simulink model "overall_model"  (R2025b)
settings: Solver=VariableStepAuto  StartTime=0.0  StopTime=10.0  RelTol=1e-3
undefined symbols (not defined in the file): mu, r0, v0
settings Model: Creator=jennaparker  LastModifiedBy=jennaparker

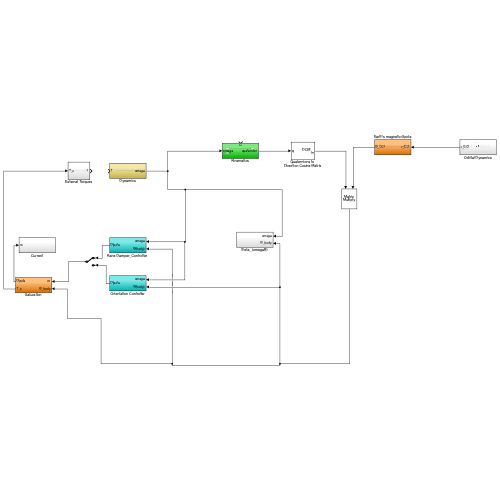
[thumbnail: Simulink's stored preview of the top-level diagram]
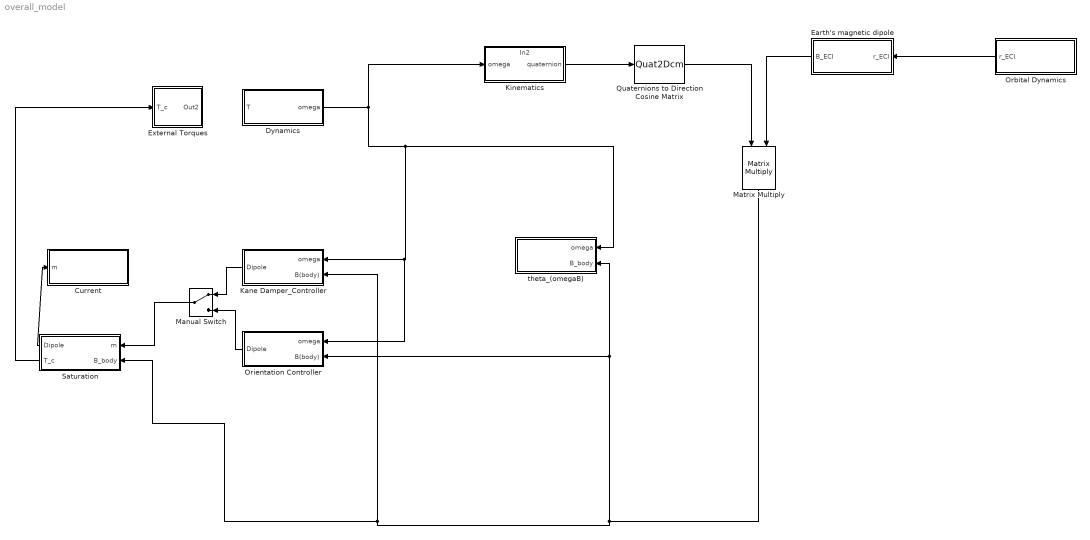
== system overall_model ==
  Current : Subsystem
  Dynamics : Subsystem
  Earth's magnetic dipole : Subsystem
  External Torques : Subsystem
  "Kane Damper_Controller " : Subsystem
  Kinematics : Subsystem
      settings: PortSchema="{\"entries\":[{\"content\":{\"sides\":[{\"content\":{\"connectorIds\":[\"In1\"]},\"type\":\"ConnectorPlacement.EquallySpacedRectSide\",\"uuid\":\"f969ea70-541e-4fe1-872d-de061585d56f\"},{\"content\":{\"connectorIds\":[\"Out1\"],\"side\":\"RIGHT\"},\"type\":\"ConnectorPlacement.EquallySpacedRectSide\",\"uuid\":\"eedb882a-61c8-46fc-b7af-f3b92c7e034c\"},{\"content\":{\"connectorIds\":[\"In2\"],\"side\":\"TOP\"},\"type\":\"ConnectorPlacement.EquallySpacedRectSide\",\"uuid\":\"40921da9-8314-4e61-b07a-c2869347cf07\"}]},\"type\":\"ConnectorPlacement.EquallySpacedConnector\",\"uuid\":\"ff868737-3a70-487e-8d9f-1b62f4bfbdd1\"}],\"packageUris\":[\"http://schema.mathworks.com/mf0/Connector/R2020b\"],\"version\":\"1.0\"}"
  Manual Switch : ManualSwitch
  Matrix Multiply : Product  Multiplication=Matrix(*)
  Orbital Dynamics : Subsystem
  Orientation Controller : Subsystem
  Quaternions to Direction Cosine Matrix : Quat2Dcm
  Saturation : Subsystem
  theta_(omegaB) : Subsystem
  wires:
  Orbital Dynamics/1(r_ECI) -> Earth's magnetic dipole/1(r_ECI)
  Earth's magnetic dipole/1(B_ECI) -> Matrix Multiply/2
  Quaternions to Direction Cosine Matrix/1 -> Matrix Multiply/1
  Kinematics/1(quaternion) -> Quaternions to Direction Cosine Matrix/1
  Dynamics/1(omega) -> Orientation Controller/1(omega), "Kane Damper_Controller "/1(omega), theta_(omegaB)/1(omega), Kinematics/1(omega)
  Saturation/1(Dipole) -> Current/1("m ")
  Saturation/2(T_c) -> External Torques/1(T_c)
  "Kane Damper_Controller "/1(Dipole) -> Manual Switch/1
  Orientation Controller/1(Dipole) -> Manual Switch/2
  Manual Switch/1 -> Saturation/1(m)
  Matrix Multiply/1 -> "Kane Damper_Controller "/2(B(body)), Saturation/2(B_body), Orientation Controller/2(B(body)), theta_(omegaB)/2(B_body)

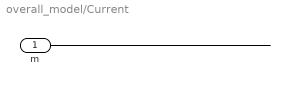
== system overall_model/Current ==
  "m " : Inport
  wires:
  "m "/1 -> ?

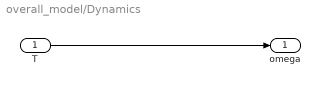
== system overall_model/Dynamics ==
  T : Inport
  omega : Outport
  wires:
  T/1 -> omega/1

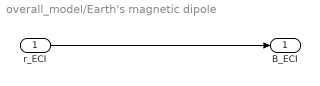
== system overall_model/Earth's magnetic dipole ==
  r_ECI : Inport
  B_ECI : Outport
  wires:
  r_ECI/1 -> B_ECI/1

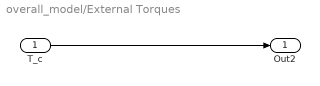
== system overall_model/External Torques ==
  T_c : Inport
  Out2 : Outport
  wires:
  T_c/1 -> Out2/1

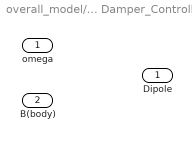
== system overall_model/Kane Damper_Controller  ==
  omega : Inport
  B(body) : Inport  Port=2
  Dipole : Outport

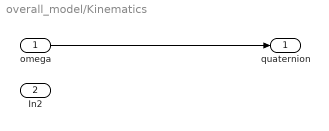
== system overall_model/Kinematics ==
  omega : Inport
  In2 : Inport  Port=2
  quaternion : Outport
  wires:
  omega/1 -> quaternion/1

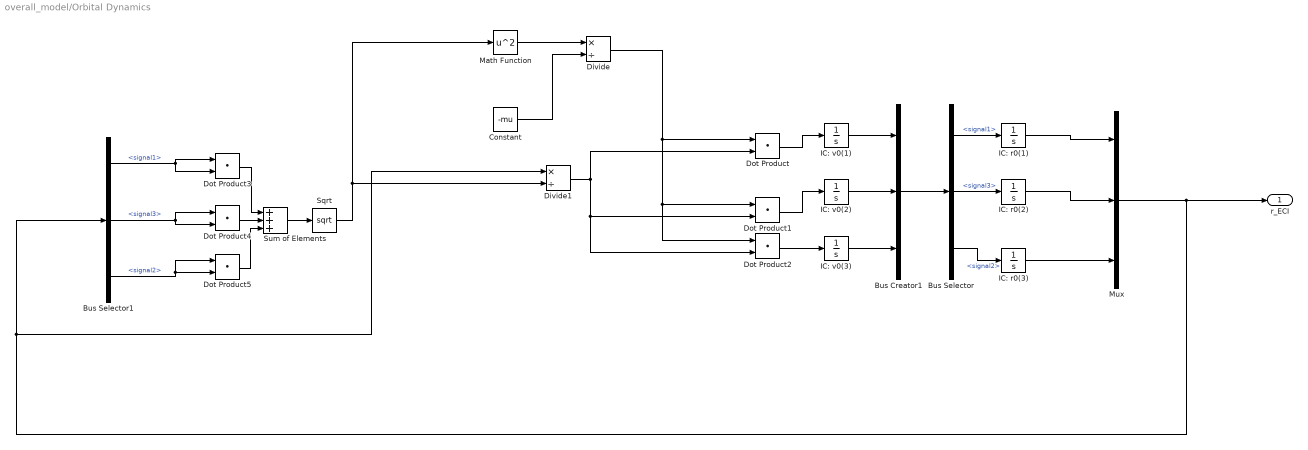
== system overall_model/Orbital Dynamics ==
  Bus Creator1 : BusCreator  Inputs=3
  Bus Selector : BusSelector  OutputSignals=signal1,signal3,signal2
  Bus Selector1 : BusSelector  OutputSignals=signal1,signal3,signal2
  Constant : Constant  Value=-mu
  Divide : Product  Inputs=*/
  Divide1 : Product  Inputs=*/
  Dot Product{,1..5} (6 alike) : DotProduct  OutDataTypeStr=Inherit: Inherit via internal rule
  IC: r0(1) : Integrator  InitialCondition=r0(1)
  IC: r0(2) : Integrator  InitialCondition=r0(2)
  IC: r0(3) : Integrator  InitialCondition=r0(3)
  IC: v0(1) : Integrator  InitialCondition=v0(1)
  IC: v0(2) : Integrator  InitialCondition=v0(2)
  IC: v0(3) : Integrator  InitialCondition=v0(3)
  Math Function : Math  Operator=square
  Mux : Mux  Inputs=3
  Sqrt : Sqrt
  Sum of Elements : Sum  Inputs=+++
  r_ECI : Outport
  wires:
  Bus Selector1/2 -> Dot Product4/1, Dot Product4/2  "<signal3>"
  Divide/1 -> Dot Product2/1, Dot Product1/1, Dot Product/1
  IC: v0(1)/1 -> Bus Creator1/1
  Bus Selector/2 -> IC: r0(2)/1  "<signal3>"
  Sum of Elements/1 -> Sqrt/1
  Dot Product/1 -> IC: v0(1)/1
  Dot Product3/1 -> Sum of Elements/1
  Bus Selector/1 -> IC: r0(1)/1  "<signal1>"
  IC: v0(3)/1 -> Bus Creator1/3
  IC: v0(2)/1 -> Bus Creator1/2
  Bus Selector1/3 -> Dot Product5/1, Dot Product5/2  "<signal2>"
  Math Function/1 -> Divide/1
  Dot Product4/1 -> Sum of Elements/2
  IC: r0(3)/1 -> Mux/3
  Mux/1 -> r_ECI/1, Divide1/1, Bus Selector1/1
  Dot Product2/1 -> IC: v0(3)/1
  Dot Product5/1 -> Sum of Elements/3
  Sqrt/1 -> Divide1/2, Math Function/1
  Bus Creator1/1 -> Bus Selector/1
  Divide1/1 -> Dot Product2/2, Dot Product1/2, Dot Product/2
  Bus Selector1/1 -> Dot Product3/2, Dot Product3/1  "<signal1>"
  Bus Selector/3 -> IC: r0(3)/1  "<signal2>"
  Dot Product1/1 -> IC: v0(2)/1
  Constant/1 -> Divide/2
  IC: r0(1)/1 -> Mux/1
  IC: r0(2)/1 -> Mux/2

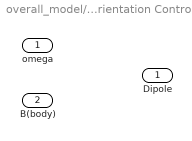
== system overall_model/Orientation Controller ==
  omega : Inport
  B(body) : Inport  Port=2
  Dipole : Outport

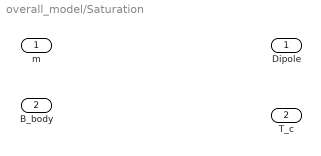
== system overall_model/Saturation ==
  m : Inport
  B_body : Inport  Port=2
  Dipole : Outport
  T_c : Outport  Port=2

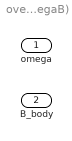
== system overall_model/theta_(omegaB) ==
  omega : Inport
  B_body : Inport  Port=2
